simulink model "PID_step"  (R2015a)
settings: Solver=ode45  StartTime=0.0  StopTime=1400.0  RelTol=1e-3
libraries: cstblocks x2, simulink x1
settings Model: Creator=Ashfaq  LastModifiedBy=Ashfaq

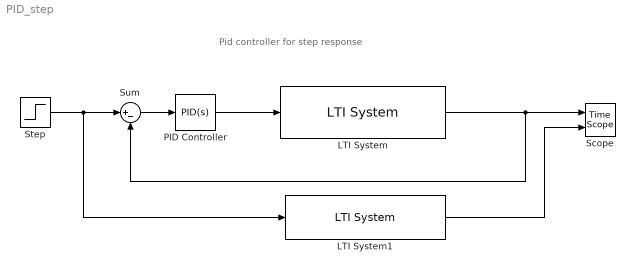
== system PID_step ==
  note: Pid controller for step response
  LTI System : cstblocks/LTI System  sys="tf([0.0003   0.0001242   0.0000024],[1   0.849   0.1274   0.0005188])"  IC=[]
  LTI System1 : cstblocks/LTI System  sys="tf([0.0003   0.0001242   0.0000024],[1   0.849   0.1274   0.0005188])"  IC=[]
  PID Controller : simulink/Continuous/PID Controller  Controller=PID  TimeDomain=Continuous-time  SampleTime=-1  IntegratorMethod=Forward Euler  FilterMethod=Forward Euler  Form=Parallel  UseFilter=on  ControllerParametersSource=internal  P=176.286602962133  I=0.909420423031738  D=-7672.31813554085  N=0.0229769673060756  InitialConditionSource=internal  InitialConditionForIntegrator=0  InitialConditionForFilter=0  ExternalReset=none  LimitOutput=off  UpperSaturationLimit=inf  LowerSaturationLimit=-inf  LinearizeAsGain=on  AntiWindupMode=none  Kb=1  TrackingMode=off  Kt=1  PParamMin=[]  PParamMax=[]  IParamMin=[]  IParamMax=[]  DParamMin=[]  DParamMax=[]  NParamMin=[]  NParamMax=[]  KbParamMin=[]  KbParamMax=[]  KtParamMin=[]  KtParamMax=[]  POutMin=[]  POutMax=[]  IOutMin=[]  IOutMax=[]  DOutMin=[]  DOutMax=[]  NOutMin=[]  NOutMax=[]  KbOutMin=[]  KbOutMax=[]  KtOutMin=[]  KtOutMax=[]  IntegratorOutMin=[]  IntegratorOutMax=[]  FilterOutMin=[]  FilterOutMax=[]  SumOutMin=[]  SumOutMax=[]  SumI1OutMin=[]  SumI1OutMax=[]  SumI2OutMin=[]  SumI2OutMax=[]  SumI3OutMin=[]  SumI3OutMax=[]  SumDOutMin=[]  SumDOutMax=[]  SaturationOutMin=[]  SaturationOutMax=[]  IntegratorContinuousStateAttributes=''  IntegratorStateMustResolveToSignalObject=off  IntegratorRTWStateStorageClass=Auto  FilterContinuousStateAttributes=''  FilterStateMustResolveToSignalObject=off  FilterRTWStateStorageClass=Auto  DifferentiatorICPrevScaledInput=0  DifferentiatorOutMin=[]  DifferentiatorOutMax=[]
  Scope : TimeScope  NumInputPorts=2
  Step : Step  SampleTime=0
  Sum : Sum  Inputs=|+-
  wires:
  Step/1 -> LTI System1/1, Sum/1
  LTI System/1 -> Scope/1, Sum/2
  Sum/1 -> PID Controller/1
  PID Controller/1 -> LTI System/1
  LTI System1/1 -> Scope/2
